simulink model "Working_MBD_UseCases"  (R2025a)
settings: Solver=FixedStepDiscrete  StartTime=0.0  StopTime=10.0  RelTol=1e-3
libraries: simulink x2
settings Model: Creator=mahij  LastModifiedBy=mahij
settings OptimizationCC: DefaultParameterBehavior=Inlined  EnhancedBackFolding=on  PassReuseOutputArgsThreshold=0.0  OptimizeBlockOrder=speed  DifferentSizesBufferReuse=on  OptimizationCustomize=off
settings DebuggingCC: ParameterTunabilityLossMsg=error
settings SFSimCC: MATLABDynamicMemAlloc=off
settings RTWCC: GenCodeOnly=on
settings CodeAppCC: ForceParamTrailComments=on  OperatorAnnotations=on

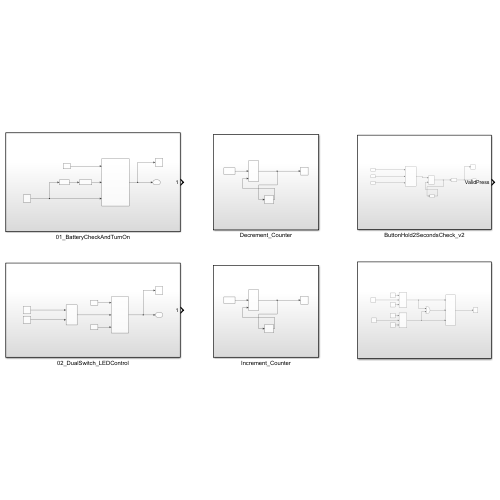
[thumbnail: Simulink's stored preview of the top-level diagram]
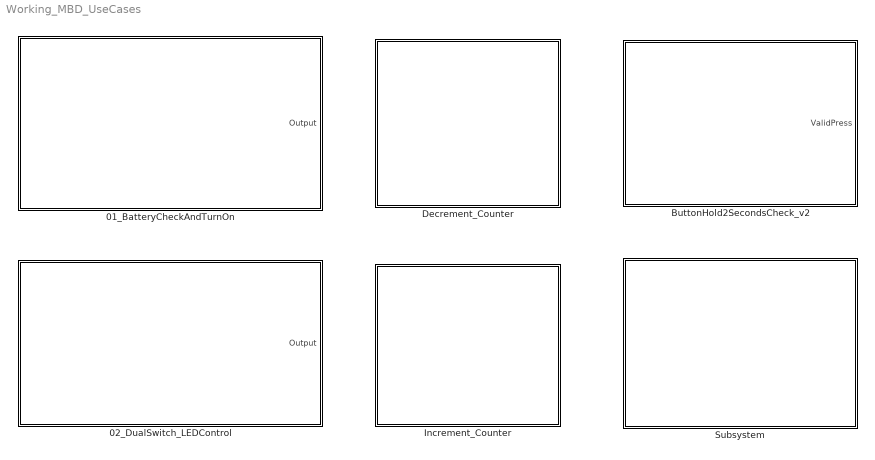
== system Working_MBD_UseCases ==
  01_BatteryCheckAndTurnOn : Subsystem
  02_DualSwitch_LEDControl : Subsystem
  ButtonHold2SecondsCheck_v2 : Subsystem
  Decrement_Counter : Subsystem
  Increment_Counter : Subsystem
  Subsystem : Subsystem

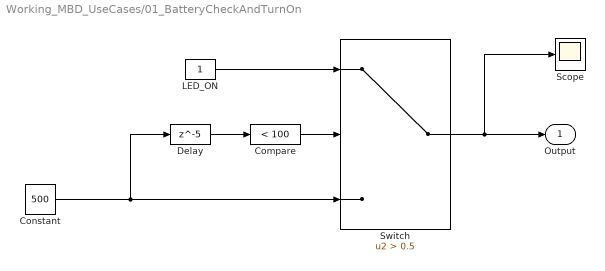
== system Working_MBD_UseCases/01_BatteryCheckAndTurnOn ==
  Compare : simulink/Logic and Bit Operations/Compare To Constant  relop=<  const=100  OutDataTypeStr=boolean
  Constant : Constant  Value=500
  Delay : Delay  DelayLength=5
  LED_ON : Constant
  Scope : Scope
      settings: ActiveDisplayYMinimum=-61.374999999999986  ActiveDisplayYMaximum=562.375
  Switch : Switch  Criteria=u2 > Threshold  Threshold=0.5  SaturateOnIntegerOverflow=off  InputSameDT=off
  Output : Outport
  wires:
  Constant/1 -> Switch/3, Delay/1
  Delay/1 -> Compare/1
  Compare/1 -> Switch/2
  LED_ON/1 -> Switch/1
  Switch/1 -> Scope/1, Output/1

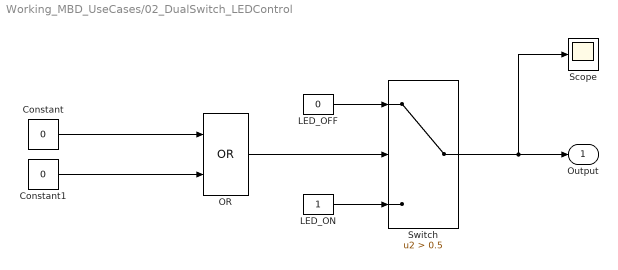
== system Working_MBD_UseCases/02_DualSwitch_LEDControl ==
  Constant : Constant  Value=0
  Constant1 : Constant  Value=0
  LED_OFF : Constant  Value=0
  LED_ON : Constant
  OR : Logic  Operator=OR  AllPortsSameDT=off  OutDataTypeStr=boolean
  Scope : Scope
      settings: ActiveDisplayYMinimum=-0.34275362318840641  ActiveDisplayYMaximum=1.2572463768115942
  Switch : Switch  Criteria=u2 > Threshold  Threshold=0.5  SaturateOnIntegerOverflow=off  InputSameDT=off
  Output : Outport
  wires:
  Constant/1 -> OR/1
  Constant1/1 -> OR/2
  OR/1 -> Switch/2
  LED_OFF/1 -> Switch/1
  LED_ON/1 -> Switch/3
  Switch/1 -> Scope/1, Output/1

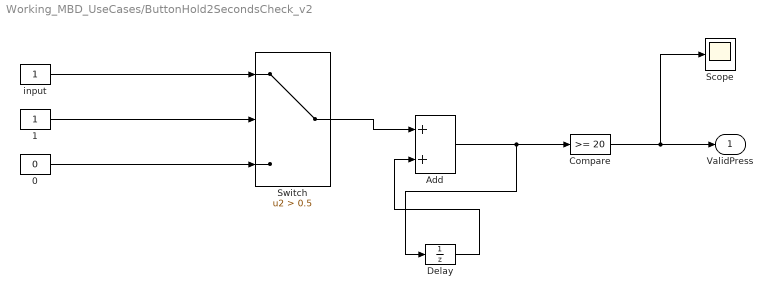
== system Working_MBD_UseCases/ButtonHold2SecondsCheck_v2 ==
  0 : Constant  Value=0
  1 : Constant
  Add : Sum
  Compare : simulink/Logic and Bit Operations/Compare To Constant  relop=>=  const=20  OutDataTypeStr=boolean
  Delay : UnitDelay  SampleTime=0.1  HasFrameUpgradeWarning=on
  Scope : Scope
      settings: ActiveDisplayYMinimum=-0.12499999999999997  ActiveDisplayYMaximum=1.125  DataLoggingVariableName=ScopeData2
  Switch : Switch  Criteria=u2 > Threshold  Threshold=0.5  SaturateOnIntegerOverflow=off  InputSameDT=off
  input : Constant
  ValidPress : Outport
  wires:
  input/1 -> Switch/1
  Delay/1 -> Add/2
  Switch/1 -> Add/1
  Add/1 -> Compare/1, Delay/1
  Compare/1 -> Scope/1, ValidPress/1
  1/1 -> Switch/2
  0/1 -> Switch/3

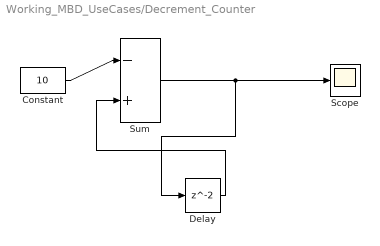
== system Working_MBD_UseCases/Decrement_Counter ==
  Constant : Constant  Value=10
  Delay : Delay
  Scope : Scope
      settings: ActiveDisplayYMinimum=-2822.5  ActiveDisplayYMaximum=302.49999999999994
  Sum : Sum  Inputs=|-+
  wires:
  Delay/1 -> Sum/2
  Sum/1 -> Delay/1, Scope/1
  Constant/1 -> Sum/1

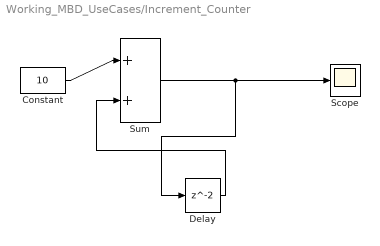
== system Working_MBD_UseCases/Increment_Counter ==
  Constant : Constant  Value=10
  Delay : Delay
  Scope : Scope
      settings: ActiveDisplayYMinimum=-2822.5  ActiveDisplayYMaximum=302.49999999999994
  Sum : Sum  Inputs=|++
  wires:
  Delay/1 -> Sum/2
  Sum/1 -> Delay/1, Scope/1
  Constant/1 -> Sum/1

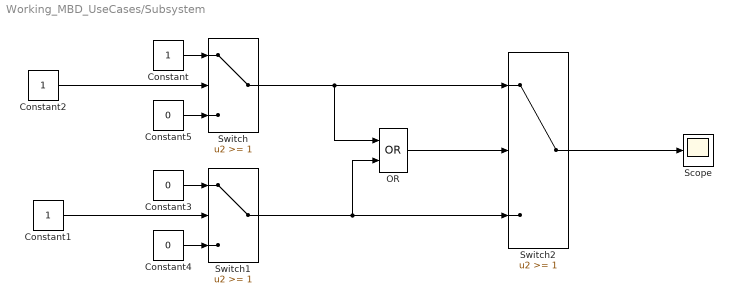
== system Working_MBD_UseCases/Subsystem ==
  Constant : Constant
  Constant1 : Constant
  Constant2 : Constant
  Constant3 : Constant  Value=0
  Constant4 : Constant  Value=0
  Constant5 : Constant  Value=0
  OR : Logic  Operator=OR  IconShape=distinctive  AllPortsSameDT=off  OutDataTypeStr=boolean
  Scope : Scope
      settings: ActiveDisplayYMinimum=-54.5011350737798  ActiveDisplayYMaximum=25.4988649262202  DataLoggingVariableName=ScopeData3
  Switch : Switch  Threshold=1  SaturateOnIntegerOverflow=off  InputSameDT=off
  Switch1 : Switch  Threshold=1  SaturateOnIntegerOverflow=off  InputSameDT=off
  Switch2 : Switch  Threshold=1  SaturateOnIntegerOverflow=off  InputSameDT=off
  wires:
  Constant2/1 -> Switch/2
  Constant1/1 -> Switch1/2
  Constant/1 -> Switch/1
  Constant3/1 -> Switch1/1
  Constant4/1 -> Switch1/3
  Constant5/1 -> Switch/3
  Switch/1 -> OR/1, Switch2/1
  Switch1/1 -> OR/2, Switch2/3
  OR/1 -> Switch2/2
  Switch2/1 -> Scope/1
